simulink model "Station"  (R2018a)
settings: Solver=VariableStepAuto  StartTime=0.0  StopTime=3600  RelTol=1e-3
undefined symbols (not defined in the file): m, n
settings Model: Creator=wass  LastModifiedBy=wass

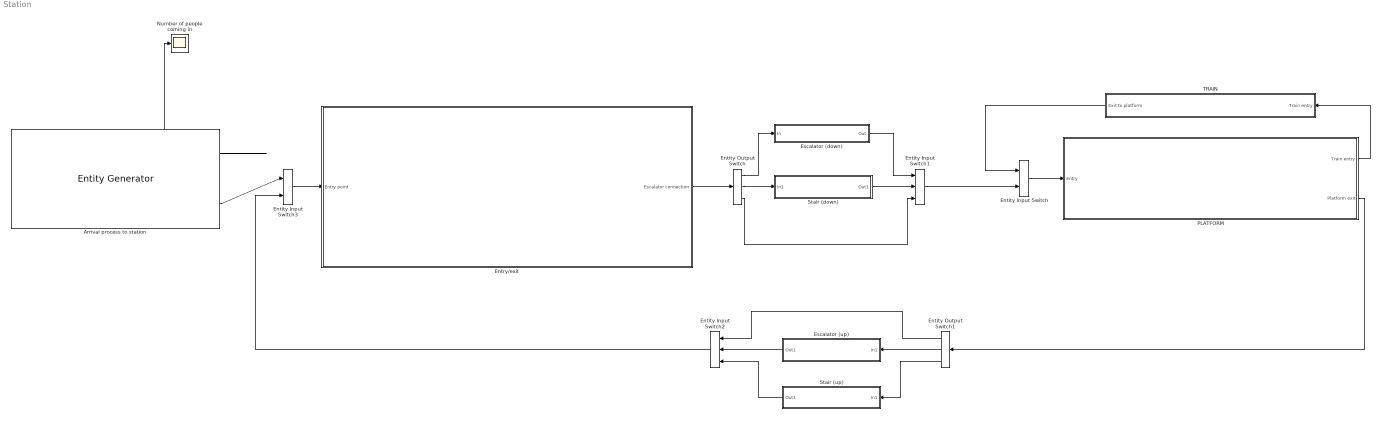
== system Station ==
  Arrival process to station : EntityGenerator  OutputPortMessageModes=n,m  TimeSource=MATLAB action  IntergenerationTimeAction=dt = poissrnd(50);  GenerateEntityAtSimulationStart=off  AttributeName=Incoming  AttributeInitialValue=2  NumberEntitiesDeparted=on  EntityType=Structured  EntityTypeName=Entity
      settings: OutputPortMap=o0,o3
  Entity Input Switch : EntityInputSwitch  InputPortMessageModes=m,m  OutputPortMessageModes=m
  Entity Input Switch1 : EntityInputSwitch  InputPortMessageModes=m,m,m  OutputPortMessageModes=m  NumberInputPorts=3
      settings: InputPortMap=u1,u2,u3
  Entity Input Switch2 : EntityInputSwitch  InputPortMessageModes=m,m,m  OutputPortMessageModes=m  NumberInputPorts=3
      settings: InputPortMap=u1,u2,u3
  Entity Input Switch3 : EntityInputSwitch  InputPortMessageModes=m,m  OutputPortMessageModes=m
  Entity Output Switch : EntityOutputSwitch  InputPortMessageModes=m  OutputPortMessageModes=m,m,m  NumberOutputPorts=3  SwitchingCriterion=Equiprobable  SwitchAttributeName=Attribute1
      settings: OutputPortMap=o0,o1,o2
  Entity Output Switch1 : EntityOutputSwitch  InputPortMessageModes=m  OutputPortMessageModes=m,m,m  NumberOutputPorts=3  SwitchAttributeName=Attribute1
      settings: OutputPortMap=o0,o1,o2
  Entry/exit : Subsystem
  Escalator (down) : Subsystem
  Escalator (up) : Subsystem
  Number of people coming in : Scope
  PLATFORM : Subsystem
  Stair (down) : Subsystem
  Stair (up) : Subsystem
  TRAIN : Subsystem
  wires:
  TRAIN/1(Exit to platform) -> Entity Input Switch/1
  Entity Input Switch/1 -> PLATFORM/1(Entry)
  Entity Output Switch/1 -> Escalator (down)/1(In)
  Entity Input Switch1/1 -> Entity Input Switch/2
  Escalator (down)/1(Out) -> Entity Input Switch1/1
  Entity Output Switch/3 -> Entity Input Switch1/3
  Entity Output Switch/2 -> Stair (down)/1(In1)
  Stair (down)/1(Out1) -> Entity Input Switch1/2
  PLATFORM/2(Platform exit) -> Entity Output Switch1/1
  Entity Output Switch1/2 -> Escalator (up)/1(In1)
  Entity Output Switch1/3 -> Stair (up)/1(In1)
  Escalator (up)/1(Out1) -> Entity Input Switch2/2
  Stair (up)/1(Out1) -> Entity Input Switch2/3
  Entity Output Switch1/1 -> Entity Input Switch2/1
  Entity Input Switch2/1 -> Entity Input Switch3/2
  Arrival process to station/2 -> Entity Input Switch3/1
  Entity Input Switch3/1 -> Entry/exit/1(Entry point)
  PLATFORM/1(Train entry) -> TRAIN/1(Train entry)
  Entry/exit/1(Escalator connection) -> Entity Output Switch/1
  Arrival process to station/1 -> Number of people coming in/1

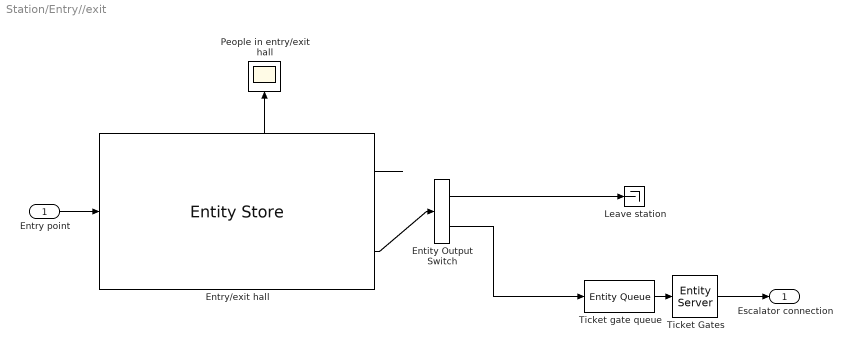
== system Station/Entry//exit ==
  Entry point : Inport
  Entity Output Switch : EntityOutputSwitch  InputPortMessageModes=m  OutputPortMessageModes=m,m  SwitchingCriterion=From attribute  SwitchAttributeName=Incoming
  Entry/exit hall : EntityStore  InputPortMessageModes=m  OutputPortMessageModes=n,m  Capacity=200  NumberEntitiesInBlock=on
      settings: OutputPortMap=o1,o4
  Leave station : Terminator
  "People in entry/exit hall " : Scope
  Ticket Gates : EntityServer  InputPortMessageModes=m  OutputPortMessageModes=m  Capacity=10  ServiceTimeValue=1
  Ticket gate queue : EntityQueue  InputPortMessageModes=m  OutputPortMessageModes=m  Capacity=inf
      settings: OutputPortMap=o5
  Escalator connection : Outport
  wires:
  Entry/exit hall/1 -> "People in entry/exit hall "/1
  Entry/exit hall/2 -> Entity Output Switch/1
  Entry point/1 -> Entry/exit hall/1
  Ticket Gates/1 -> Escalator connection/1
  Ticket gate queue/1 -> Ticket Gates/1
  Entity Output Switch/2 -> Ticket gate queue/1
  Entity Output Switch/1 -> Leave station/1

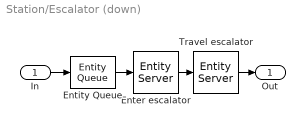
== system Station/Escalator (down) ==
  In : Inport
  Enter escalator : EntityServer  InputPortMessageModes=m  OutputPortMessageModes=m  Capacity=1  ServiceTimeValue=1
  Entity Queue : EntityQueue  InputPortMessageModes=m  OutputPortMessageModes=m  Capacity=inf
      settings: OutputPortMap=o5
  Travel escalator : EntityServer  InputPortMessageModes=m  OutputPortMessageModes=m  Capacity=inf  ServiceTimeValue=20
  Out : Outport
  wires:
  In/1 -> Entity Queue/1
  Enter escalator/1 -> Travel escalator/1
  Travel escalator/1 -> Out/1
  Entity Queue/1 -> Enter escalator/1

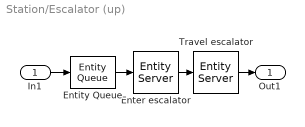
== system Station/Escalator (up) ==
  In1 : Inport
  Enter escalator : EntityServer  InputPortMessageModes=m  OutputPortMessageModes=m  Capacity=1  ServiceTimeValue=1
  Entity Queue : EntityQueue  InputPortMessageModes=m  OutputPortMessageModes=m  Capacity=inf
      settings: OutputPortMap=o5
  Travel escalator : EntityServer  InputPortMessageModes=m  OutputPortMessageModes=m  Capacity=inf  ServiceTimeValue=40
  Out1 : Outport
  wires:
  In1/1 -> Entity Queue/1
  Enter escalator/1 -> Travel escalator/1
  Travel escalator/1 -> Out1/1
  Entity Queue/1 -> Enter escalator/1

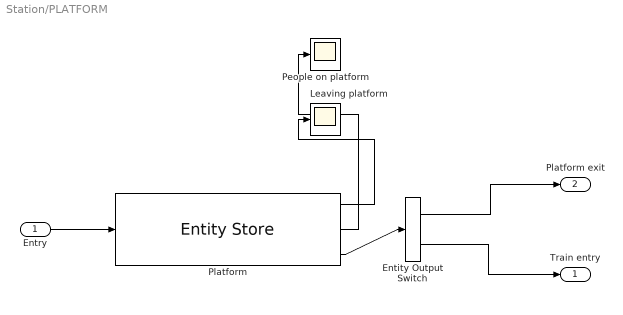
== system Station/PLATFORM ==
  Entry : Inport
  Entity Output Switch : EntityOutputSwitch  InputPortMessageModes=m  OutputPortMessageModes=m,m  SwitchingCriterion=From attribute  SwitchAttributeName=Incoming
  "Leaving platform " : Scope
  People on platform : Scope
  "Platform " : EntityStore  InputPortMessageModes=m  OutputPortMessageModes=n,n,m  Capacity=500  NumberEntitiesDeparted=on  NumberEntitiesInBlock=on
      settings: OutputPortMap=o0,o1,o4
  Train entry : Outport
  Platform exit : Outport  Port=2
  wires:
  "Platform "/2 -> People on platform/1
  "Platform "/1 -> "Leaving platform "/1
  Entry/1 -> "Platform "/1
  "Platform "/3 -> Entity Output Switch/1
  Entity Output Switch/1 -> Platform exit/1
  Entity Output Switch/2 -> Train entry/1

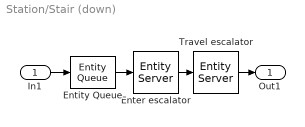
== system Station/Stair (down) ==
  In1 : Inport
  Enter escalator : EntityServer  InputPortMessageModes=m  OutputPortMessageModes=m  Capacity=1  ServiceTimeValue=1
  Entity Queue : EntityQueue  InputPortMessageModes=m  OutputPortMessageModes=m  Capacity=inf
      settings: OutputPortMap=o5
  Travel escalator : EntityServer  InputPortMessageModes=m  OutputPortMessageModes=m  Capacity=inf  ServiceTimeValue=40
  Out1 : Outport
  wires:
  In1/1 -> Entity Queue/1
  Enter escalator/1 -> Travel escalator/1
  Travel escalator/1 -> Out1/1
  Entity Queue/1 -> Enter escalator/1

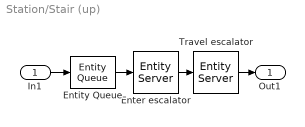
== system Station/Stair (up) ==
  In1 : Inport
  Enter escalator : EntityServer  InputPortMessageModes=m  OutputPortMessageModes=m  Capacity=1  ServiceTimeValue=1
  Entity Queue : EntityQueue  InputPortMessageModes=m  OutputPortMessageModes=m  Capacity=inf
      settings: OutputPortMap=o5
  Travel escalator : EntityServer  InputPortMessageModes=m  OutputPortMessageModes=m  Capacity=inf  ServiceTimeValue=40
  Out1 : Outport
  wires:
  In1/1 -> Entity Queue/1
  Enter escalator/1 -> Travel escalator/1
  Travel escalator/1 -> Out1/1
  Entity Queue/1 -> Enter escalator/1

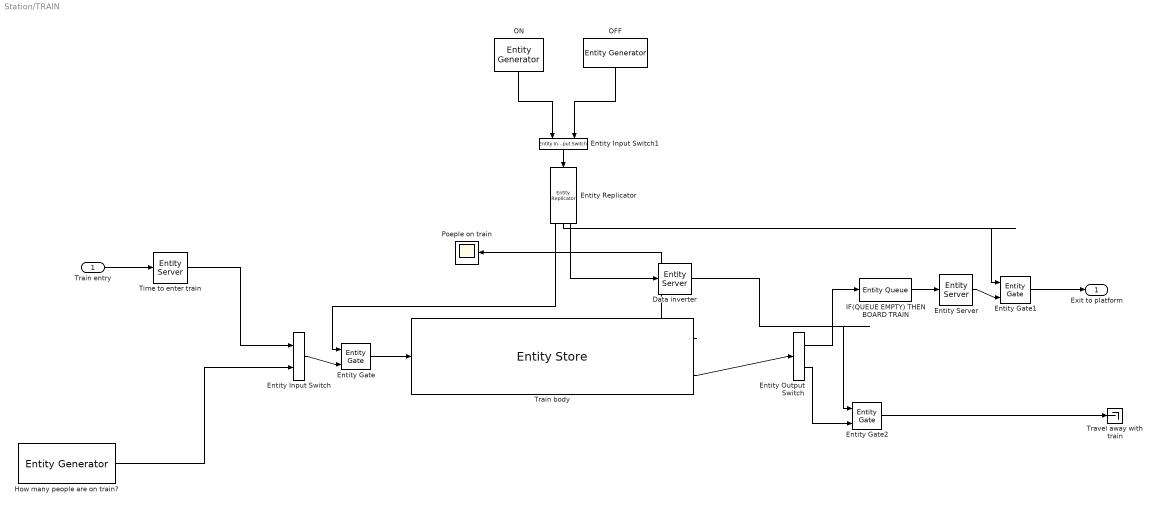
== system Station/TRAIN ==
  Train entry : Inport
  Data inverter : EntityServer  InputPortMessageModes=m  OutputPortMessageModes=m  Capacity=inf  ServiceTimeValue=0  EntryAction=entity = 1 - entity
  Entity Input Switch : EntityInputSwitch  InputPortMessageModes=m,m  OutputPortMessageModes=m
  Entity Input Switch1 : EntityInputSwitch  InputPortMessageModes=m,m  OutputPortMessageModes=m
  Entity Output Switch : EntityOutputSwitch  InputPortMessageModes=m  OutputPortMessageModes=m,m  SwitchingCriterion=From attribute  SwitchAttributeName=Incoming
  Entity Gate : EntityGate  InputPortMessageModes=m,m  OutputPortMessageModes=m
  Entity Gate1 : EntityGate  InputPortMessageModes=m,m  OutputPortMessageModes=m
  Entity Gate2 : EntityGate  InputPortMessageModes=m,m  OutputPortMessageModes=m
  Entity Replicator : EntityReplicator  InputPortMessageModes=m  OutputPortMessageModes=m,m,m  NumberReplicas=2  HoldOriginalEntityUntilAllReplicasDepart=on
      settings: OutputPortMap=o0,o1,o2
  Entity Server : EntityServer  InputPortMessageModes=m  OutputPortMessageModes=m  Capacity=1  ServiceTimeValue=1
  "How many people are on train? " : EntityGenerator  OutputPortMessageModes=m  TimeSource=MATLAB action  IntergenerationTimeAction=|  GenerateEntityAtSimulationStart=off  GenerateAction=|  AttributeName=Incoming  EntityType=Structured  EntityTypeName=Entity
      IntergenerationTimeAction=|
      | persistent entity_number
      | 
      | people_per_wave = 100
      | train_periodicity = 16*60
      | 
      | if isempty(entity_number)
      |     entity_number = 1
      | end
      | 
      | if entity_number == 1
      |     dt = train_periodicity - 60
      | 
      | elseif mod(entity_number, people_per_wave) == 1
      |     dt = train_periodicity
      | else
      |     dt = 0
      | end
      |     
      |         
      |     
      |     
      | entity_number = entity_number + 1
      GenerateAction=|
      | prob_incoming = 0.1
      | 
      | entity.Incoming = 1 + (rand() > prob_incoming)
  IF(QUEUE EMPTY) THEN BOARD TRAIN : EntityQueue  InputPortMessageModes=m  OutputPortMessageModes=m
      settings: OutputPortMap=o5
  OFF : EntityGenerator  OutputPortMessageModes=m  Period=16*60  IntergenerationTimeAction=dt = 5;  GenerateEntityAtSimulationStart=off  AttributeName=entity  AttributeInitialValue=0  EntityTypeName=Entity
  ON : EntityGenerator  OutputPortMessageModes=m  TimeSource=MATLAB action  Period=5  IntergenerationTimeAction=|  GenerateEntityAtSimulationStart=off  AttributeName=entity  EntityTypeName=Entity  DataInitialValue=1
      | persistent first
      | if isempty(first)
      |     first = true;
      |     dt = 15*60; 
      | else
      |     dt = 16*60;
      | end
  Poeple on train : Scope
  Time to enter train : EntityServer  InputPortMessageModes=m  OutputPortMessageModes=m  Capacity=1  ServiceTimeSource=MATLAB action  ServiceTimeAction=|
      | % Time to enter train should depend on how
      | % many people are leaving / staying on the train
      | dt = 1;
  Train body : EntityStore  InputPortMessageModes=m  OutputPortMessageModes=n,m  Capacity=200  NumberEntitiesInBlock=on
      settings: OutputPortMap=o1,o4
  Travel away with train : Terminator
  Exit to platform : Outport
  wires:
  ON/1 -> Entity Input Switch1/1
  OFF/1 -> Entity Input Switch1/2
  "How many people are on train? "/1 -> Entity Input Switch/2
  Train entry/1 -> Time to enter train/1
  Time to enter train/1 -> Entity Input Switch/1
  Entity Output Switch/1 -> IF(QUEUE EMPTY) THEN BOARD TRAIN/1
  Entity Gate1/1 -> Exit to platform/1
  Entity Gate/1 -> Train body/1
  Entity Input Switch/1 -> Entity Gate/2
  Entity Input Switch1/1 -> Entity Replicator/1
  Entity Replicator/1 -> Entity Gate/1
  Entity Replicator/2 -> Entity Gate1/1
  IF(QUEUE EMPTY) THEN BOARD TRAIN/1 -> Entity Server/1
  Train body/2 -> Entity Output Switch/1
  Entity Output Switch/2 -> Entity Gate2/2
  Entity Replicator/3 -> Data inverter/1
  Data inverter/1 -> Entity Gate2/1
  Train body/1 -> Poeple on train/1
  Entity Gate2/1 -> Travel away with train/1
  Entity Server/1 -> Entity Gate1/2
